simulink model "LinearModelClosedLoopTest_RW_and_Mgt_models"  (R2023a)
settings: Solver=VariableStepAuto  StartTime=0.0  StopTime=500  RelTol=1e-3
values from neighbouring files (symbols this model uses):
  A = [A11 zeros(3) A13 ... (first row only)    [State_Space_SC.m]
  B = (1/438)*(60/(2*pi))*1e-3    (= 2.18020469989e-05)    [State_Space_RW.m]    (also in State_Space_SC.m = [I^-1 I^-1 I^-1)
  I = 1e-7*[336109.715 0 0 ... (first row only)    [State_Space_SC.m]
  J = J_rotor+ J_flywheel    (= 7.1569e-05)    [State_Space_RW.m]
  Ke = (1/1120)*(60/(2*pi))    (= 0.00852615766564)    [State_Space_RW.m]
  Kt = 8.55e-3    (= 0.00855)    [State_Space_RW.m]
  La = 0.222e-3    (= 0.000222)    [State_Space_RW.m]
  Ra = 3.36    [State_Space_RW.m]
  T_ext = 6.850e-7    (= 6.85e-07)    [State_Space_RW.m]
  T_max = 7.7501e-3    (= 0.0077501)    [State_Space_RW.m]
undefined symbols (not defined in the file or in its folder): A_model, B_model, C_model, D_model, n_cal, R_mgt, T_max_mgt
libraries: matrix_library x9, slpidlib x6, simulink_extras x3, vrlib x2, aerolibutil x1
settings Model: Creator=Personal  LastModifiedBy=Personal

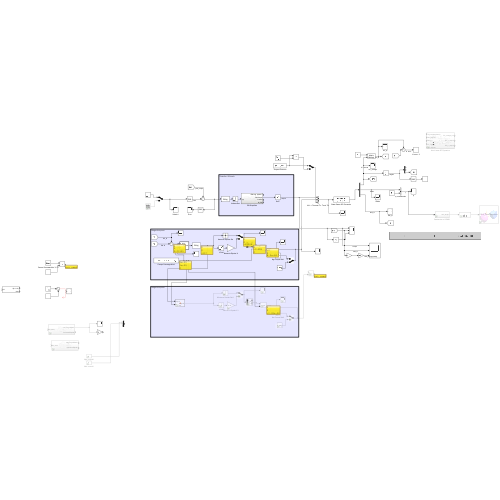
[thumbnail: Simulink's stored preview of the top-level diagram]
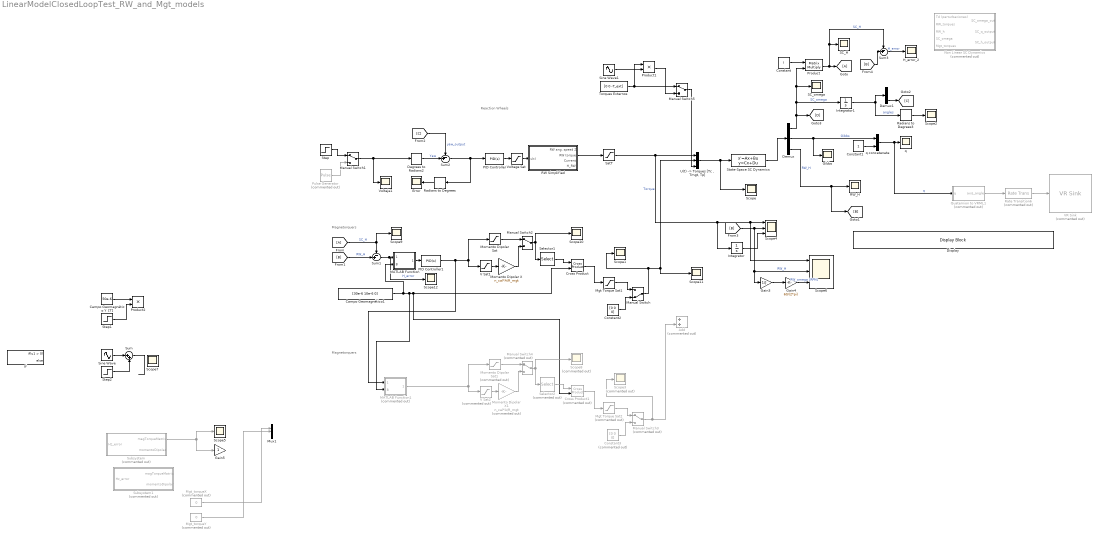
== system LinearModelClosedLoopTest_RW_and_Mgt_models ==
  note: Reaction Wheels
  note: Magnetorquers
  note: Magnetorquers
  Add : Sum  Commented=on
  Campo Geomagnético Y  [T] : Constant  Value=50e-6
  Campo Geomagnético1 : Constant  Value=[30e-6 10e-6 0]
  Constant : Constant  Value=I
  Constant1 : Constant
  Constant2 : Constant  Value=[0 0 0]
  Constant3 : Constant  Commented=on  Value=[0 0 0]
  Cross Product : matrix_library/Cross Product
  Cross Product1 : matrix_library/Cross Product  Commented=on
  Degrees to Radians2 : simulink_extras/Transformations/Degrees to Radians
  Demux : Demux  Outputs=3
  Demux1 : Demux  Outputs=3
  Display : DisplayBlock  LabelPosition=Hide  Transparency=1
  Error : Scope
  From : From
  Gain3 : Gain  Gain=1/J
  Gain4 : Gain  Gain=60/(2*pi)
  Gain5 : Gain
  Gibbs : Scope
  Goto : Goto
  H_error_2 : Scope
  If : If
  Integrator : Integrator
  Integrator1 : Integrator  InitialCondition=[0 0 0]
  MATLAB Function : MATLAB Function  TreatAsAtomicUnit=on
  MATLAB Function1 : MATLAB Function  Commented=on  TreatAsAtomicUnit=on
  Manual Switch : ManualSwitch  CurrentSetting=0
  Manual Switch1 : ManualSwitch
  Manual Switch2 : ManualSwitch
  Manual Switch3 : ManualSwitch  Commented=on
  Manual Switch4 : ManualSwitch  Commented=on
  Manual Switch5 : ManualSwitch
  Mgt Torque Sat1 : Saturate  UpperLimit=T_max_mgt  LowerLimit=-T_max_mgt
  Mgt Torque Sat2 : Saturate  Commented=on  UpperLimit=T_max_mgt  LowerLimit=-T_max_mgt
  Mgt_torqueX : Constant  Commented=on  Value=0
  Mgt_torqueY : Constant  Commented=on  Value=0
  Momento Dipolar Sat : Saturate  UpperLimit=(5/R_mgt)*A*n_cal  LowerLimit=-(5/R_mgt)*A*n_cal
  Momento Dipolar Sat1 : Saturate  Commented=on  UpperLimit=(5/R_mgt)*A*n_cal  LowerLimit=-(5/R_mgt)*A*n_cal
  Momento Dipolar X : Gain  Gain=n_cal*A/R_mgt
  Momento Dipolar X1 : Gain  Commented=on  Gain=n_cal*A/R_mgt
  Mux1 : Mux  Inputs=3
  Non Linear SC Dynamics : Subsystem  Commented=on
  PID Controller : slpidlib/PID Controller  Controller=PID  Form=Parallel  TimeDomain=Continuous-time  UseExternalTs=off  SampleTime=-1  IntegratorMethod=Forward Euler  FilterMethod=Forward Euler  ControllerParametersSource=internal  P=4500  I=800  UseKiTs=off  D=8000  N=100  UseFilter=on  TunerSelectOption=Transfer Function Based (PID Tuner App)  InitialConditionSource=internal  InitialConditionForIntegrator=0  InitialConditionForFilter=0  DifferentiatorICPrevScaledInput=0  ExternalReset=none  TrackingMode=off  Kt=1  LimitOutput=off  SatLimitsSource=internal  UpperSaturationLimit=1  LowerSaturationLimit=-1  LinearizeAsGain=on  AntiWindupMode=none  Kb=1  LimitIntegrator=off  UpperIntegratorSaturationLimit=inf  LowerIntegratorSaturationLimit=-inf  POutMin=[]  POutMax=[]  IOutMin=[]  IOutMax=[]  DOutMin=[]  DOutMax=[]  NOutMin=[]  NOutMax=[]  SumOutMin=[]  SumOutMax=[]  SaturationOutMin=[]  SaturationOutMax=[]  PParamMin=[]  PParamMax=[]  IParamMin=[]  IParamMax=[]  DParamMin=[]  DParamMax=[]  NParamMin=[]  NParamMax=[]  KbParamMin=[]  KbParamMax=[]  KtParamMin=[]  KtParamMax=[]  KbOutMin=[]  KbOutMax=[]  KtOutMin=[]  KtOutMax=[]  IntegratorOutMin=[]  IntegratorOutMax=[]  FilterOutMin=[]  FilterOutMax=[]  SumI1OutMin=[]  SumI1OutMax=[]  SumI2OutMin=[]  SumI2OutMax=[]  SumI3OutMin=[]  SumI3OutMax=[]  SumI4OutMin=[]  SumI4OutMax=[]  SumDOutMin=[]  SumDOutMax=[]  DifferentiatorOutMin=[]  DifferentiatorOutMax=[]  FilterDiffOutCoefMin=[]  FilterDiffOutCoefMax=[]  ReciprocalOutMin=[]  ReciprocalOutMax=[]  SumDenOutMin=[]  SumDenOutMax=[]  SumNumOutMin=[]  SumNumOutMax=[]  DivideOutMin=[]  DivideOutMax=[]  UdiffTsProdOutMin=[]  UdiffTsProdOutMax=[]  NTsProdOutMin=[]  NTsProdOutMax=[]  UintegralTsProdOutMin=[]  UintegralTsProdOutMax=[]  UngainTsProdOutMin=[]  UngainTsProdOutMax=[]  ClampingZeroOutDataTypeStr=Inherit: Inherit via back propagation  ClampingZeroOutMin=[]  ClampingZeroOutMax=[]  FilterDenConstantOutDataTypeStr=Inherit: Inherit via back propagation  FilterDenConstantOutMin=[]  FilterDenConstantOutMax=[]  PCopyOutDataTypeStr=Inherit: Inherit via back propagation  PCopyOutMin=[]  PCopyOutMax=[]  NCopyOutDataTypeStr=Inherit: Inherit via back propagation  NCopyOutMin=[]  NCopyOutMax=[]  IntegratorContinuousStateAttributes=''  IntegratorStateMustResolveToSignalObject=off  IntegratorRTWStateStorageClass=Auto  FilterContinuousStateAttributes=''  FilterStateMustResolveToSignalObject=off  FilterRTWStateStorageClass=Auto  ParallelPVariant=InternalParameters  IdealPVariant=Disabled  IVariant=InternalParameters  DVariant=InternalParameters  IntegratorVariant=Continuous  SatVariant=Disabled  AWVariant=Passthrough  PCopyVariant=Disabled  TRVariant=Disabled  FdbkBlocksVariant=Forward  IdealPFdbkVariant=Disabled  SatFdbkVariant=Disabled  DerivativeFilterVariant=ContFilter  NVariant=InternalParameters  NCopyVariant=Disabled  FilterICVariant=InternalICsFilter  IntegratorICVariant=InternalICs  ExternalResetVariant=Disabled  TRSumVariant=Passthrough  SumFdbkVariant=Disabled  SumVariant=Sum_PID  TsampFilterVariant=InternalTs  TsampNgainVariant=Passthrough  TsampIntegralVariant=Disabled_SignalSpec  ExternalSaturationOutDataTypeStr=Inherit: Same as second input
  PID Controller1 : slpidlib/PID Controller  Controller=PID  Form=Parallel  TimeDomain=Continuous-time  UseExternalTs=off  SampleTime=-1  IntegratorMethod=Forward Euler  FilterMethod=Forward Euler  ControllerParametersSource=internal  P=4500  I=800  UseKiTs=off  D=8000  N=100  UseFilter=on  TunerSelectOption=Transfer Function Based (PID Tuner App)  InitialConditionSource=internal  InitialConditionForIntegrator=0  InitialConditionForFilter=0  DifferentiatorICPrevScaledInput=0  ExternalReset=none  TrackingMode=off  Kt=1  LimitOutput=off  SatLimitsSource=internal  UpperSaturationLimit=1  LowerSaturationLimit=-1  LinearizeAsGain=on  AntiWindupMode=none  Kb=1  LimitIntegrator=off  UpperIntegratorSaturationLimit=inf  LowerIntegratorSaturationLimit=-inf  POutMin=[]  POutMax=[]  IOutMin=[]  IOutMax=[]  DOutMin=[]  DOutMax=[]  NOutMin=[]  NOutMax=[]  SumOutMin=[]  SumOutMax=[]  SaturationOutMin=[]  SaturationOutMax=[]  PParamMin=[]  PParamMax=[]  IParamMin=[]  IParamMax=[]  DParamMin=[]  DParamMax=[]  NParamMin=[]  NParamMax=[]  KbParamMin=[]  KbParamMax=[]  KtParamMin=[]  KtParamMax=[]  KbOutMin=[]  KbOutMax=[]  KtOutMin=[]  KtOutMax=[]  IntegratorOutMin=[]  IntegratorOutMax=[]  FilterOutMin=[]  FilterOutMax=[]  SumI1OutMin=[]  SumI1OutMax=[]  SumI2OutMin=[]  SumI2OutMax=[]  SumI3OutMin=[]  SumI3OutMax=[]  SumI4OutMin=[]  SumI4OutMax=[]  SumDOutMin=[]  SumDOutMax=[]  DifferentiatorOutMin=[]  DifferentiatorOutMax=[]  FilterDiffOutCoefMin=[]  FilterDiffOutCoefMax=[]  ReciprocalOutMin=[]  ReciprocalOutMax=[]  SumDenOutMin=[]  SumDenOutMax=[]  SumNumOutMin=[]  SumNumOutMax=[]  DivideOutMin=[]  DivideOutMax=[]  UdiffTsProdOutMin=[]  UdiffTsProdOutMax=[]  NTsProdOutMin=[]  NTsProdOutMax=[]  UintegralTsProdOutMin=[]  UintegralTsProdOutMax=[]  UngainTsProdOutMin=[]  UngainTsProdOutMax=[]  ClampingZeroOutDataTypeStr=Inherit: Inherit via back propagation  ClampingZeroOutMin=[]  ClampingZeroOutMax=[]  FilterDenConstantOutDataTypeStr=Inherit: Inherit via back propagation  FilterDenConstantOutMin=[]  FilterDenConstantOutMax=[]  PCopyOutDataTypeStr=Inherit: Inherit via back propagation  PCopyOutMin=[]  PCopyOutMax=[]  NCopyOutDataTypeStr=Inherit: Inherit via back propagation  NCopyOutMin=[]  NCopyOutMax=[]  IntegratorContinuousStateAttributes=''  IntegratorStateMustResolveToSignalObject=off  IntegratorRTWStateStorageClass=Auto  FilterContinuousStateAttributes=''  FilterStateMustResolveToSignalObject=off  FilterRTWStateStorageClass=Auto  ParallelPVariant=InternalParameters  IdealPVariant=Disabled  IVariant=InternalParameters  DVariant=InternalParameters  IntegratorVariant=Continuous  SatVariant=Disabled  AWVariant=Passthrough  PCopyVariant=Disabled  TRVariant=Disabled  FdbkBlocksVariant=Forward  IdealPFdbkVariant=Disabled  SatFdbkVariant=Disabled  DerivativeFilterVariant=ContFilter  NVariant=InternalParameters  NCopyVariant=Disabled  FilterICVariant=InternalICsFilter  IntegratorICVariant=InternalICs  ExternalResetVariant=Disabled  TRSumVariant=Passthrough  SumFdbkVariant=Disabled  SumVariant=Sum_PID  TsampFilterVariant=InternalTs  TsampNgainVariant=Passthrough  TsampIntegralVariant=Disabled_SignalSpec  ExternalSaturationOutDataTypeStr=Inherit: Same as second input
  Product : Product  Multiplication=Matrix(*)
  Product1 : Product
  Product2 : Product
  Pulse Generator : DiscretePulseGenerator  Commented=on  PulseType=Time based  Amplitude=45  Period=50  PulseWidth=50
  Quaternion to VRML1 : Subsystem  Commented=on
  RW Simplified : Subsystem
  RW_H : Scope
  Radians to Degrees : simulink_extras/Transformations/Radians to Degrees
  Radians to Degrees3 : simulink_extras/Transformations/Radians to Degrees
  Rate Transition6 : RateTransition  Commented=on
  SC_H : Scope
  SC_omega : Scope
  SatT : Saturate  UpperLimit=T_max  LowerLimit=-T_max
  Scope{,1..2,5,7,9..12} (9 alike) : Scope
  Scope3 : Scope  Commented=on
  Scope4 : Scope  NumInputPorts=3
  Scope6 : Scope  NumInputPorts=3
  Scope8 : Scope  Commented=on
  Selector1 : Selector  InputPortWidth=3  IndexOptions=Index vector (dialog)  Indices=[1 3 2]  OutputSizes=1
  Selector2 : Selector  Commented=on  InputPortWidth=3  IndexOptions=Index vector (dialog)  Indices=[3 1 2]  OutputSizes=1
  Sine Wave : Sin  Amplitude=3e-6  Frequency=0.1  SampleTime=0
  Sine Wave1 : Sin  Frequency=0.05  SampleTime=0
  "State-Space SC Dynamics " : StateSpace  A=A_model  B=B_model  C=C_model  D=D_model  InitialCondition=0
  Step : Step  Time=5  After=90  SampleTime=0
  Step1 : Step  Time=0  SampleTime=0
  Step2 : Step  Time=0  After=40e-6  SampleTime=0
  Subsystem : Subsystem  Commented=on
  Subsystem1 : Subsystem  Commented=on
  Sum : Sum  Inputs=|++
  Sum1 : Sum  Inputs=-+|
  Sum2 : Sum  Inputs=-+|
  Sum3 : Sum  Inputs=-+|
  Torques Externos : Constant  Value=[0 0 -T_ext]
  "U(t) -> Torques [Tc , Tmgt, Tp]" : Concatenate  NumInputs=3
  V Sat1 : Saturate  UpperLimit=5  LowerLimit=-5
  V Sat2 : Saturate  Commented=on  UpperLimit=5  LowerLimit=-5
  VR Sink : vrlib/VR Sink  Commented=on  InstantiateOnLoad=on  SampleTime=0.1  ViewEnable=on  RemoteChange=off  RemoteView=off  FieldsWritten=STLB_Transform.rotation.4.1.1.double  WorldFileName=EscenarioCubeSat.x3d  AutoView=off  VideoDimensions=[]  AllowVariableSize=off
  Voltage Sat : Saturate  UpperLimit=6  LowerLimit=-6
  Voltaje1 : Scope
  q : Scope
  q concatenate : Concatenate
  wires:
  Pulse Generator/1 -> Manual Switch1/2
  Degrees to Radians2/1 -> Sum2/2  "Yaw"
  Manual Switch1/1 -> Voltaje1/1, Degrees to Radians2/1
  Step/1 -> Manual Switch1/1
  "State-Space SC Dynamics "/1 -> Demux/1
  "U(t) -> Torques [Tc , Tmgt, Tp]"/1 -> Scope/1, "State-Space SC Dynamics "/1
  Demux/1 -> [D], Integrator1/1, Product/2, SC_omega/1  "SC_omega"
  Demux/2 -> q concatenate/1, Gibbs/1  "Gibbs"
  Demux/3 -> [B], RW_H/1  "RW_H"
  Sum2/1 -> Radians to Degrees/1, PID Controller/1
  SatT/1 -> Integrator/1, Scope6/1, Scope4/1, "U(t) -> Torques [Tc , Tmgt, Tp]"/1  "Torque"
  Torques Externos/1 -> Product1/1, Manual Switch5/1
  Subsystem/1(magTorqueMatrix) -> Scope5/1, Gain5/1
  Constant/1 -> Product/1
  Product/1 -> Sum3/1, SC_H/1, Goto/1  "SC_H"
  From/1 -> Sum1/1, Scope9/1  "SC_H"
  [B] -> Sum1/2  "RW_H"
  Sum1/1 -> Scope12/1, MATLAB Function/1("H_error ")  "H_error"
  Integrator1/1 -> Demux1/1, Radians to Degrees3/1  "angles"
  Demux1/3 -> [C]
  Radians to Degrees3/1 -> Scope2/1
  [C] -> Sum2/1  "yaw_output"
  Radians to Degrees/1 -> Error/1
  [B] -> Gain3/1, Scope6/2, Scope4/2  "RW_H"
  Integrator/1 -> Scope4/3
  Constant1/1 -> q concatenate/2
  q concatenate/1 -> Quaternion to VRML1/1(q), q/1  "q"
  Rate Transition6/1 -> VR Sink/1
  Quaternion to VRML1/1(axis_angle) -> Rate Transition6/1
  Gain3/1 -> Gain4/1
  Gain4/1 -> Scope6/3  "RW_omega [RPM]"
  RW Simplified/2(RW torque) -> SatT/1
  PID Controller/1 -> Voltage Sat/1
  Voltage Sat/1 -> RW Simplified/1(v(t))
  Mgt_torqueY/1 -> Mux1/2
  Mgt_torqueX/1 -> Mux1/1
  Mgt Torque Sat1/1 -> Manual Switch/1
  [B] -> Sum3/2
  Sum3/1 -> H_error_2/1  "H_error"
  V Sat1/1 -> Momento Dipolar X/1
  Momento Dipolar X/1 -> Manual Switch2/2
  Campo Geomagnético Y  [T]/1 -> Product2/1
  Step1/1 -> Product2/2
  Sine Wave/1 -> Sum/1
  Step2/1 -> Sum/2
  Sum/1 -> ?
  Momento Dipolar Sat/1 -> Manual Switch2/1
  MATLAB Function/1(H_error) -> PID Controller1/1
  Manual Switch2/1 -> Selector1/1, Scope10/1
  Campo Geomagnético1/1 -> MATLAB Function1/2(B), Cross Product1/2, Cross Product/2, MATLAB Function/2(B)
  Manual Switch/1 -> "U(t) -> Torques [Tc , Tmgt, Tp]"/2, Scope11/1, Scope1/1
  Selector1/1 -> Cross Product/1
  Cross Product/1 -> Mgt Torque Sat1/1
  PID Controller1/1 -> MATLAB Function1/1("signal "), Momento Dipolar Sat/1, V Sat1/1
  Constant2/1 -> Manual Switch/2
  Constant3/1 -> Manual Switch3/2
  MATLAB Function1/1(signal) -> V Sat2/1, Momento Dipolar Sat1/1
  Cross Product1/1 -> Mgt Torque Sat2/1
  Selector2/1 -> Cross Product1/1
  Manual Switch3/1 -> Scope3/1, Add/2
  Manual Switch4/1 -> Scope8/1, Selector2/1
  Momento Dipolar Sat1/1 -> Manual Switch4/1
  Momento Dipolar X1/1 -> Manual Switch4/2
  V Sat2/1 -> Momento Dipolar X1/1
  Mgt Torque Sat2/1 -> Manual Switch3/1
  Sine Wave1/1 -> Product1/2
  Manual Switch5/1 -> "U(t) -> Torques [Tc , Tmgt, Tp]"/3
  Product1/1 -> Manual Switch5/2

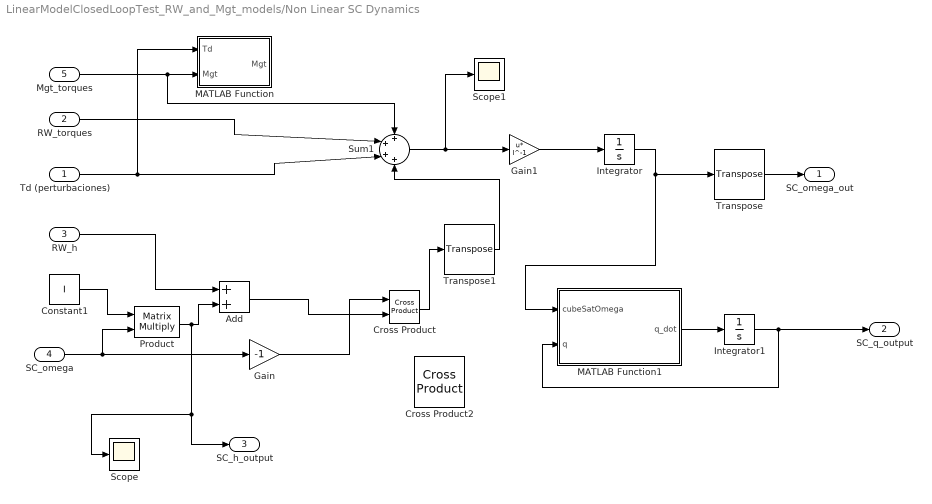
== system LinearModelClosedLoopTest_RW_and_Mgt_models/Non Linear SC Dynamics ==
  Td (perturbaciones) : Inport
  RW_torques : Inport  Port=2
  RW_h : Inport  Port=3
  SC_omega : Inport  Port=4
  Mgt_torques : Inport  Port=5
  Add : Sum
  Constant1 : Constant  Value=I
  Cross Product : vrlib/Utilities/Cross Product
  Cross Product2 : matrix_library/Cross Product
  Gain : Gain  Gain=-1
  Gain1 : Gain  Gain=I^-1  Multiplication=Matrix(u*K)
  Integrator : Integrator  InitialCondition=[0 0 0]
  Integrator1 : Integrator  InitialCondition=[0 0 0 1]
  MATLAB Function : MATLAB Function  TreatAsAtomicUnit=on
  MATLAB Function1 : MATLAB Function  TreatAsAtomicUnit=on
  Product : Product  Multiplication=Matrix(*)
  Scope : Scope
  Scope1 : Scope
  Sum1 : Sum  Inputs=++++
  Transpose : matrix_library/Transpose
  Transpose1 : matrix_library/Transpose
  SC_omega_out : Outport
  SC_q_output : Outport  Port=2
  SC_h_output : Outport  Port=3
  wires:
  RW_torques/1 -> Sum1/2
  Td (perturbaciones)/1 -> MATLAB Function/1(Td), Sum1/3
  Integrator1/1 -> MATLAB Function1/2(q), SC_q_output/1
  Constant1/1 -> Product/1
  Product/1 -> Scope/1, SC_h_output/1, Add/2
  RW_h/1 -> Add/1
  Gain/1 -> Cross Product/1
  Add/1 -> Cross Product/2
  Cross Product/1 -> Transpose1/1
  Sum1/1 -> Scope1/1, Gain1/1
  Gain1/1 -> Integrator/1
  Integrator/1 -> MATLAB Function1/1(cubeSatOmega), Transpose/1
  MATLAB Function1/1(q_dot) -> Integrator1/1
  SC_omega/1 -> Product/2, Gain/1
  Transpose/1 -> SC_omega_out/1
  Transpose1/1 -> Sum1/4
  Mgt_torques/1 -> Sum1/1, MATLAB Function/2("Mgt ")

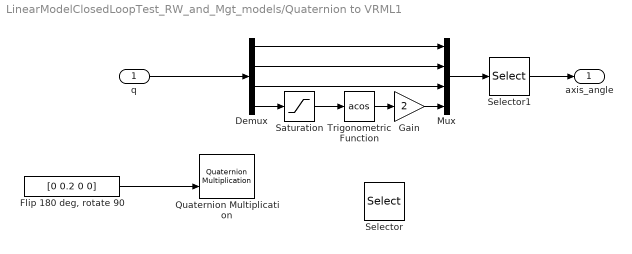
== system LinearModelClosedLoopTest_RW_and_Mgt_models/Quaternion to VRML1 ==
  q : Inport
  Demux : Demux
  "Flip 180 deg, rotate 90" : Constant  Value=[0 0.2 0 0]
  Gain : Gain  Gain=2
  Mux : Mux
  Quaternion Multiplication : aerolibutil/Quaternion Multiplication
  Saturation : Saturate  UpperLimit=1  LowerLimit=-1  ZeroCross=off
  Selector : Selector  InputPortWidth=3  IndexOptions=Index vector (dialog)  Indices=[1 3]  OutputSizes=1
  Selector1 : Selector  InputPortWidth=4  IndexOptions=Index vector (dialog)  Indices=[2 3 1 4]  OutputSizes=1
  Trigonometric Function : Trigonometry  Operator=acos
  axis_angle : Outport  VectorParamsAs1DForOutWhenUnconnected=off
  wires:
  Demux/2 -> Mux/2
  "Flip 180 deg, rotate 90"/1 -> Quaternion Multiplication/2
  q/1 -> Demux/1
  Demux/1 -> Mux/1
  Mux/1 -> Selector1/1
  Selector1/1 -> axis_angle/1
  Trigonometric Function/1 -> Gain/1
  Gain/1 -> Mux/4
  Demux/3 -> Mux/3
  Saturation/1 -> Trigonometric Function/1
  Demux/4 -> Saturation/1

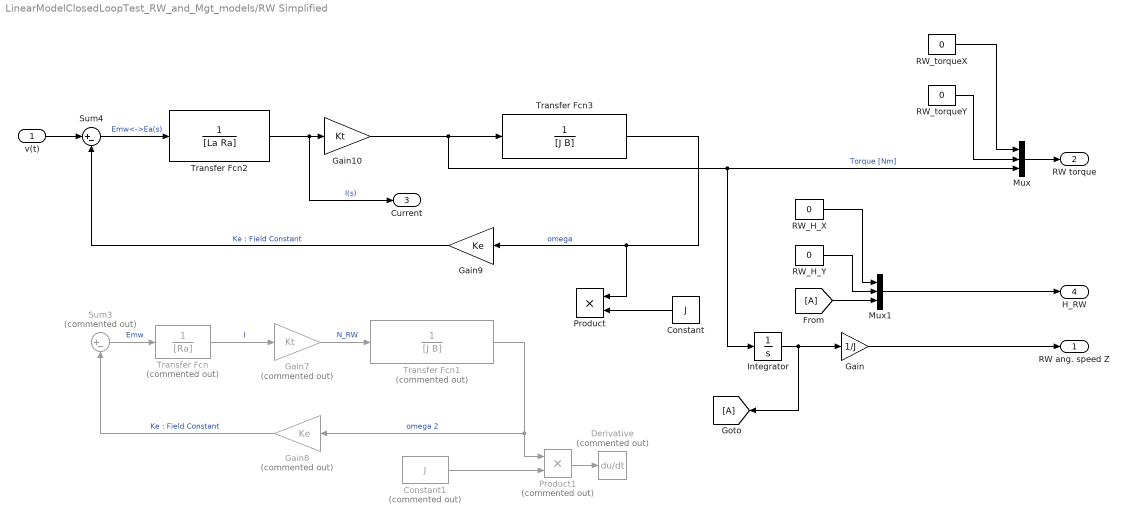
== system LinearModelClosedLoopTest_RW_and_Mgt_models/RW Simplified ==
  v(t) : Inport
  Constant : Constant  Value=J
  Constant1 : Constant  Commented=on  Value=J
  Derivative : Derivative  Commented=on
  From : From
  Gain : Gain  Gain=1/J
  Gain10 : Gain  Gain=Kt
  Gain7 : Gain  Commented=on  Gain=Kt
  Gain8 : Gain  Commented=on  Gain=Ke
  Gain9 : Gain  Gain=Ke
  Goto : Goto
  Integrator : Integrator
  Mux : Mux  Inputs=3
  Mux1 : Mux  Inputs=3
  Product : Product
  Product1 : Product  Commented=on
  RW_H_X : Constant  Value=0
  RW_H_Y : Constant  Value=0
  RW_torqueX : Constant  Value=0
  RW_torqueY : Constant  Value=0
  Sum3 : Sum  Commented=on  Inputs=|+-
  Sum4 : Sum  Inputs=|+-
  Transfer Fcn : TransferFcn  Commented=on  Denominator=[Ra]
  Transfer Fcn1 : TransferFcn  Commented=on  Denominator=[J B]
  Transfer Fcn2 : TransferFcn  Denominator=[La Ra]
  Transfer Fcn3 : TransferFcn  Denominator=[J B]
  RW ang. speed Z : Outport  VectorParamsAs1DForOutWhenUnconnected=off
  RW torque : Outport  Port=2  VectorParamsAs1DForOutWhenUnconnected=off
  Current : Outport  Port=3  VectorParamsAs1DForOutWhenUnconnected=off
  H_RW : Outport  Port=4  VectorParamsAs1DForOutWhenUnconnected=off
  wires:
  Transfer Fcn2/1 -> Current/1, Gain10/1  "I(s)"
  Sum4/1 -> Transfer Fcn2/1  "Emw<->Ea(s)"
  Gain9/1 -> Sum4/2  "Ke : Field Constant"
  Transfer Fcn3/1 -> Gain9/1, Product/1  "omega"
  Constant/1 -> Product/2
  Integrator/1 -> Goto/1, Gain/1
  v(t)/1 -> Sum4/1
  Product1/1 -> Derivative/1
  Constant1/1 -> Product1/2
  Transfer Fcn1/1 -> Product1/1, Gain8/1  "omega 2"
  Gain7/1 -> Transfer Fcn1/1  "N_RW"
  Sum3/1 -> Transfer Fcn/1  "Emw"
  Transfer Fcn/1 -> Gain7/1  "I"
  Gain8/1 -> Sum3/2  "Ke : Field Constant"
  RW_H_X/1 -> Mux1/1
  RW_H_Y/1 -> Mux1/2
  Mux1/1 -> H_RW/1
  RW_torqueX/1 -> Mux/1
  RW_torqueY/1 -> Mux/2
  Mux/1 -> RW torque/1
  Gain10/1 -> Integrator/1, Mux/3, Transfer Fcn3/1  "Torque [Nm]"
  Gain/1 -> RW ang. speed Z/1
  From/1 -> Mux1/3

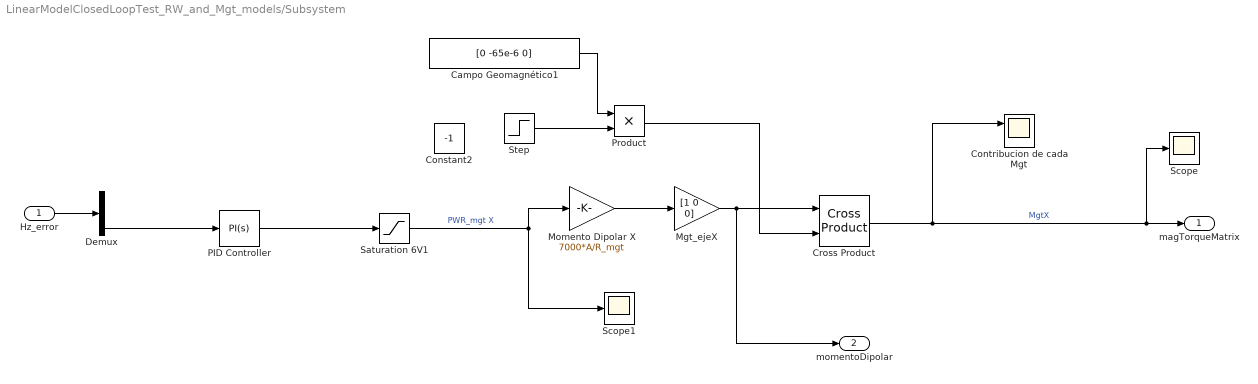
== system LinearModelClosedLoopTest_RW_and_Mgt_models/Subsystem ==
  Hz_error : Inport
  Campo Geomagnético1 : Constant  Value=[0 -65e-6 0]
  Constant2 : Constant  Value=-1
  Contribucion de cada Mgt : Scope  NumInputPorts=2
  Cross Product : matrix_library/Cross Product
  Demux : Demux  Outputs=3
  Mgt_ejeX : Gain  Gain=[1 0 0]
  Momento Dipolar X : Gain  Gain=7000*A/R_mgt
  PID Controller : slpidlib/PID Controller  Controller=PI  Form=Parallel  TimeDomain=Continuous-time  UseExternalTs=off  SampleTime=-1  IntegratorMethod=Forward Euler  FilterMethod=Forward Euler  ControllerParametersSource=internal  P=1  I=1  UseKiTs=off  D=0  N=100  UseFilter=on  TunerSelectOption=Transfer Function Based (PID Tuner App)  InitialConditionSource=internal  InitialConditionForIntegrator=0  InitialConditionForFilter=0  DifferentiatorICPrevScaledInput=0  ExternalReset=none  TrackingMode=off  Kt=1  LimitOutput=off  SatLimitsSource=internal  UpperSaturationLimit=inf  LowerSaturationLimit=-inf  LinearizeAsGain=on  AntiWindupMode=none  Kb=1  LimitIntegrator=off  UpperIntegratorSaturationLimit=inf  LowerIntegratorSaturationLimit=-inf  POutMin=[]  POutMax=[]  IOutMin=[]  IOutMax=[]  DOutMin=[]  DOutMax=[]  NOutMin=[]  NOutMax=[]  SumOutMin=[]  SumOutMax=[]  SaturationOutMin=[]  SaturationOutMax=[]  PParamMin=[]  PParamMax=[]  IParamMin=[]  IParamMax=[]  DParamMin=[]  DParamMax=[]  NParamMin=[]  NParamMax=[]  KbParamMin=[]  KbParamMax=[]  KtParamMin=[]  KtParamMax=[]  KbOutMin=[]  KbOutMax=[]  KtOutMin=[]  KtOutMax=[]  IntegratorOutMin=[]  IntegratorOutMax=[]  FilterOutMin=[]  FilterOutMax=[]  SumI1OutMin=[]  SumI1OutMax=[]  SumI2OutMin=[]  SumI2OutMax=[]  SumI3OutMin=[]  SumI3OutMax=[]  SumI4OutMin=[]  SumI4OutMax=[]  SumDOutMin=[]  SumDOutMax=[]  DifferentiatorOutMin=[]  DifferentiatorOutMax=[]  FilterDiffOutCoefMin=[]  FilterDiffOutCoefMax=[]  ReciprocalOutMin=[]  ReciprocalOutMax=[]  SumDenOutMin=[]  SumDenOutMax=[]  SumNumOutMin=[]  SumNumOutMax=[]  DivideOutMin=[]  DivideOutMax=[]  UdiffTsProdOutMin=[]  UdiffTsProdOutMax=[]  NTsProdOutMin=[]  NTsProdOutMax=[]  UintegralTsProdOutMin=[]  UintegralTsProdOutMax=[]  UngainTsProdOutMin=[]  UngainTsProdOutMax=[]  ClampingZeroOutDataTypeStr=Inherit: Inherit via back propagation  ClampingZeroOutMin=[]  ClampingZeroOutMax=[]  FilterDenConstantOutDataTypeStr=Inherit: Inherit via back propagation  FilterDenConstantOutMin=[]  FilterDenConstantOutMax=[]  PCopyOutDataTypeStr=Inherit: Inherit via back propagation  PCopyOutMin=[]  PCopyOutMax=[]  NCopyOutDataTypeStr=Inherit: Inherit via back propagation  NCopyOutMin=[]  NCopyOutMax=[]  IntegratorContinuousStateAttributes=''  IntegratorStateMustResolveToSignalObject=off  IntegratorRTWStateStorageClass=Auto  FilterContinuousStateAttributes=''  FilterStateMustResolveToSignalObject=off  FilterRTWStateStorageClass=Auto  ParallelPVariant=InternalParameters  IdealPVariant=Disabled  IVariant=InternalParameters  DVariant=Disabled  IntegratorVariant=Continuous  SatVariant=Disabled  AWVariant=Passthrough  PCopyVariant=Disabled  TRVariant=Disabled  FdbkBlocksVariant=Forward  IdealPFdbkVariant=Disabled  SatFdbkVariant=Disabled  DerivativeFilterVariant=Disabled  NVariant=Disabled  NCopyVariant=Disabled_SignalSpec  FilterICVariant=Disabled  IntegratorICVariant=InternalICs  ExternalResetVariant=Disabled  TRSumVariant=Passthrough  SumFdbkVariant=Disabled  SumVariant=Sum_PI  TsampFilterVariant=InternalTs  TsampNgainVariant=Passthrough  TsampIntegralVariant=Disabled_SignalSpec  ExternalSaturationOutDataTypeStr=Inherit: Same as second input
  Product : Product
  Saturation 6V1 : Saturate  UpperLimit=10  LowerLimit=-10
  Scope : Scope
  Scope1 : Scope
  Step : Step  Time=0  After=-1  SampleTime=0
  magTorqueMatrix : Outport
  momentoDipolar : Outport  Port=2
  wires:
  Saturation 6V1/1 -> Momento Dipolar X/1, Scope1/1  "PWR_mgt X"
  Hz_error/1 -> Demux/1
  Product/1 -> Cross Product/2
  PID Controller/1 -> Saturation 6V1/1
  Momento Dipolar X/1 -> Mgt_ejeX/1
  Cross Product/1 -> Contribucion de cada Mgt/1, Scope/1, magTorqueMatrix/1  "MgtX"
  Mgt_ejeX/1 -> momentoDipolar/1, Cross Product/1
  Campo Geomagnético1/1 -> Product/1
  Step/1 -> Product/2
  Demux/3 -> PID Controller/1

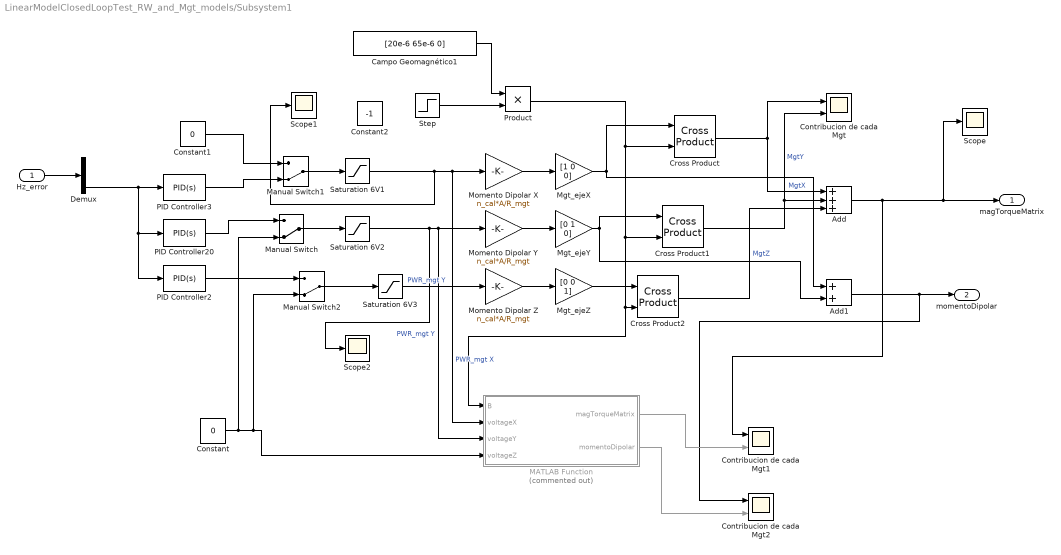
== system LinearModelClosedLoopTest_RW_and_Mgt_models/Subsystem1 ==
  Hz_error : Inport
  Add : Sum  Inputs=+++
  Add1 : Sum
  Campo Geomagnético1 : Constant  Value=[20e-6 65e-6 0]
  Constant : Constant  Value=0
  Constant1 : Constant  Value=0
  Constant2 : Constant  Value=-1
  Contribucion de cada Mgt : Scope  NumInputPorts=2
  Contribucion de cada Mgt1 : Scope  NumInputPorts=2
  Contribucion de cada Mgt2 : Scope  NumInputPorts=2
  Cross Product : matrix_library/Cross Product
  Cross Product1 : matrix_library/Cross Product
  Cross Product2 : matrix_library/Cross Product
  Demux : Demux  Outputs=3
  MATLAB Function : MATLAB Function  Commented=on  TreatAsAtomicUnit=on
  Manual Switch : ManualSwitch  CurrentSetting=0
  Manual Switch1 : ManualSwitch  CurrentSetting=0
  Manual Switch2 : ManualSwitch  CurrentSetting=0
  Mgt_ejeX : Gain  Gain=[1 0 0]
  Mgt_ejeY : Gain  Gain=[0 1 0]
  Mgt_ejeZ : Gain  Gain=[0 0 1]
  Momento Dipolar X : Gain  Gain=n_cal*A/R_mgt
  Momento Dipolar Y : Gain  Gain=n_cal*A/R_mgt
  Momento Dipolar Z : Gain  Gain=n_cal*A/R_mgt
  PID Controller2 : slpidlib/PID Controller  Controller=PID  Form=Parallel  TimeDomain=Continuous-time  UseExternalTs=off  SampleTime=-1  IntegratorMethod=Forward Euler  FilterMethod=Forward Euler  ControllerParametersSource=internal  P=4500  I=800  UseKiTs=off  D=8000  N=100  UseFilter=on  TunerSelectOption=Transfer Function Based (PID Tuner App)  InitialConditionSource=internal  InitialConditionForIntegrator=0  InitialConditionForFilter=0  DifferentiatorICPrevScaledInput=0  ExternalReset=none  TrackingMode=off  Kt=1  LimitOutput=off  SatLimitsSource=internal  UpperSaturationLimit=1  LowerSaturationLimit=-1  LinearizeAsGain=on  AntiWindupMode=none  Kb=1  LimitIntegrator=off  UpperIntegratorSaturationLimit=inf  LowerIntegratorSaturationLimit=-inf  POutMin=[]  POutMax=[]  IOutMin=[]  IOutMax=[]  DOutMin=[]  DOutMax=[]  NOutMin=[]  NOutMax=[]  SumOutMin=[]  SumOutMax=[]  SaturationOutMin=[]  SaturationOutMax=[]  PParamMin=[]  PParamMax=[]  IParamMin=[]  IParamMax=[]  DParamMin=[]  DParamMax=[]  NParamMin=[]  NParamMax=[]  KbParamMin=[]  KbParamMax=[]  KtParamMin=[]  KtParamMax=[]  KbOutMin=[]  KbOutMax=[]  KtOutMin=[]  KtOutMax=[]  IntegratorOutMin=[]  IntegratorOutMax=[]  FilterOutMin=[]  FilterOutMax=[]  SumI1OutMin=[]  SumI1OutMax=[]  SumI2OutMin=[]  SumI2OutMax=[]  SumI3OutMin=[]  SumI3OutMax=[]  SumI4OutMin=[]  SumI4OutMax=[]  SumDOutMin=[]  SumDOutMax=[]  DifferentiatorOutMin=[]  DifferentiatorOutMax=[]  FilterDiffOutCoefMin=[]  FilterDiffOutCoefMax=[]  ReciprocalOutMin=[]  ReciprocalOutMax=[]  SumDenOutMin=[]  SumDenOutMax=[]  SumNumOutMin=[]  SumNumOutMax=[]  DivideOutMin=[]  DivideOutMax=[]  UdiffTsProdOutMin=[]  UdiffTsProdOutMax=[]  NTsProdOutMin=[]  NTsProdOutMax=[]  UintegralTsProdOutMin=[]  UintegralTsProdOutMax=[]  UngainTsProdOutMin=[]  UngainTsProdOutMax=[]  ClampingZeroOutDataTypeStr=Inherit: Inherit via back propagation  ClampingZeroOutMin=[]  ClampingZeroOutMax=[]  FilterDenConstantOutDataTypeStr=Inherit: Inherit via back propagation  FilterDenConstantOutMin=[]  FilterDenConstantOutMax=[]  PCopyOutDataTypeStr=Inherit: Inherit via back propagation  PCopyOutMin=[]  PCopyOutMax=[]  NCopyOutDataTypeStr=Inherit: Inherit via back propagation  NCopyOutMin=[]  NCopyOutMax=[]  IntegratorContinuousStateAttributes=''  IntegratorStateMustResolveToSignalObject=off  IntegratorRTWStateStorageClass=Auto  FilterContinuousStateAttributes=''  FilterStateMustResolveToSignalObject=off  FilterRTWStateStorageClass=Auto  ParallelPVariant=InternalParameters  IdealPVariant=Disabled  IVariant=InternalParameters  DVariant=InternalParameters  IntegratorVariant=Continuous  SatVariant=Disabled  AWVariant=Passthrough  PCopyVariant=Disabled  TRVariant=Disabled  FdbkBlocksVariant=Forward  IdealPFdbkVariant=Disabled  SatFdbkVariant=Disabled  DerivativeFilterVariant=ContFilter  NVariant=InternalParameters  NCopyVariant=Disabled  FilterICVariant=InternalICsFilter  IntegratorICVariant=InternalICs  ExternalResetVariant=Disabled  TRSumVariant=Passthrough  SumFdbkVariant=Disabled  SumVariant=Sum_PID  TsampFilterVariant=InternalTs  TsampNgainVariant=Passthrough  TsampIntegralVariant=Disabled_SignalSpec  ExternalSaturationOutDataTypeStr=Inherit: Same as second input
  PID Controller20 : slpidlib/PID Controller  Controller=PID  Form=Parallel  TimeDomain=Continuous-time  UseExternalTs=off  SampleTime=-1  IntegratorMethod=Forward Euler  FilterMethod=Forward Euler  ControllerParametersSource=internal  P=4500  I=800  UseKiTs=off  D=8000  N=100  UseFilter=on  TunerSelectOption=Transfer Function Based (PID Tuner App)  InitialConditionSource=internal  InitialConditionForIntegrator=0  InitialConditionForFilter=0  DifferentiatorICPrevScaledInput=0  ExternalReset=none  TrackingMode=off  Kt=1  LimitOutput=off  SatLimitsSource=internal  UpperSaturationLimit=1  LowerSaturationLimit=-1  LinearizeAsGain=on  AntiWindupMode=none  Kb=1  LimitIntegrator=off  UpperIntegratorSaturationLimit=inf  LowerIntegratorSaturationLimit=-inf  POutMin=[]  POutMax=[]  IOutMin=[]  IOutMax=[]  DOutMin=[]  DOutMax=[]  NOutMin=[]  NOutMax=[]  SumOutMin=[]  SumOutMax=[]  SaturationOutMin=[]  SaturationOutMax=[]  PParamMin=[]  PParamMax=[]  IParamMin=[]  IParamMax=[]  DParamMin=[]  DParamMax=[]  NParamMin=[]  NParamMax=[]  KbParamMin=[]  KbParamMax=[]  KtParamMin=[]  KtParamMax=[]  KbOutMin=[]  KbOutMax=[]  KtOutMin=[]  KtOutMax=[]  IntegratorOutMin=[]  IntegratorOutMax=[]  FilterOutMin=[]  FilterOutMax=[]  SumI1OutMin=[]  SumI1OutMax=[]  SumI2OutMin=[]  SumI2OutMax=[]  SumI3OutMin=[]  SumI3OutMax=[]  SumI4OutMin=[]  SumI4OutMax=[]  SumDOutMin=[]  SumDOutMax=[]  DifferentiatorOutMin=[]  DifferentiatorOutMax=[]  FilterDiffOutCoefMin=[]  FilterDiffOutCoefMax=[]  ReciprocalOutMin=[]  ReciprocalOutMax=[]  SumDenOutMin=[]  SumDenOutMax=[]  SumNumOutMin=[]  SumNumOutMax=[]  DivideOutMin=[]  DivideOutMax=[]  UdiffTsProdOutMin=[]  UdiffTsProdOutMax=[]  NTsProdOutMin=[]  NTsProdOutMax=[]  UintegralTsProdOutMin=[]  UintegralTsProdOutMax=[]  UngainTsProdOutMin=[]  UngainTsProdOutMax=[]  ClampingZeroOutDataTypeStr=Inherit: Inherit via back propagation  ClampingZeroOutMin=[]  ClampingZeroOutMax=[]  FilterDenConstantOutDataTypeStr=Inherit: Inherit via back propagation  FilterDenConstantOutMin=[]  FilterDenConstantOutMax=[]  PCopyOutDataTypeStr=Inherit: Inherit via back propagation  PCopyOutMin=[]  PCopyOutMax=[]  NCopyOutDataTypeStr=Inherit: Inherit via back propagation  NCopyOutMin=[]  NCopyOutMax=[]  IntegratorContinuousStateAttributes=''  IntegratorStateMustResolveToSignalObject=off  IntegratorRTWStateStorageClass=Auto  FilterContinuousStateAttributes=''  FilterStateMustResolveToSignalObject=off  FilterRTWStateStorageClass=Auto  ParallelPVariant=InternalParameters  IdealPVariant=Disabled  IVariant=InternalParameters  DVariant=InternalParameters  IntegratorVariant=Continuous  SatVariant=Disabled  AWVariant=Passthrough  PCopyVariant=Disabled  TRVariant=Disabled  FdbkBlocksVariant=Forward  IdealPFdbkVariant=Disabled  SatFdbkVariant=Disabled  DerivativeFilterVariant=ContFilter  NVariant=InternalParameters  NCopyVariant=Disabled  FilterICVariant=InternalICsFilter  IntegratorICVariant=InternalICs  ExternalResetVariant=Disabled  TRSumVariant=Passthrough  SumFdbkVariant=Disabled  SumVariant=Sum_PID  TsampFilterVariant=InternalTs  TsampNgainVariant=Passthrough  TsampIntegralVariant=Disabled_SignalSpec  ExternalSaturationOutDataTypeStr=Inherit: Same as second input
  PID Controller3 : slpidlib/PID Controller  Controller=PID  Form=Parallel  TimeDomain=Continuous-time  UseExternalTs=off  SampleTime=-1  IntegratorMethod=Forward Euler  FilterMethod=Forward Euler  ControllerParametersSource=internal  P=4500  I=800  UseKiTs=off  D=8000  N=100  UseFilter=on  TunerSelectOption=Transfer Function Based (PID Tuner App)  InitialConditionSource=internal  InitialConditionForIntegrator=0  InitialConditionForFilter=0  DifferentiatorICPrevScaledInput=0  ExternalReset=none  TrackingMode=off  Kt=1  LimitOutput=off  SatLimitsSource=internal  UpperSaturationLimit=1  LowerSaturationLimit=-1  LinearizeAsGain=on  AntiWindupMode=none  Kb=1  LimitIntegrator=off  UpperIntegratorSaturationLimit=inf  LowerIntegratorSaturationLimit=-inf  POutMin=[]  POutMax=[]  IOutMin=[]  IOutMax=[]  DOutMin=[]  DOutMax=[]  NOutMin=[]  NOutMax=[]  SumOutMin=[]  SumOutMax=[]  SaturationOutMin=[]  SaturationOutMax=[]  PParamMin=[]  PParamMax=[]  IParamMin=[]  IParamMax=[]  DParamMin=[]  DParamMax=[]  NParamMin=[]  NParamMax=[]  KbParamMin=[]  KbParamMax=[]  KtParamMin=[]  KtParamMax=[]  KbOutMin=[]  KbOutMax=[]  KtOutMin=[]  KtOutMax=[]  IntegratorOutMin=[]  IntegratorOutMax=[]  FilterOutMin=[]  FilterOutMax=[]  SumI1OutMin=[]  SumI1OutMax=[]  SumI2OutMin=[]  SumI2OutMax=[]  SumI3OutMin=[]  SumI3OutMax=[]  SumI4OutMin=[]  SumI4OutMax=[]  SumDOutMin=[]  SumDOutMax=[]  DifferentiatorOutMin=[]  DifferentiatorOutMax=[]  FilterDiffOutCoefMin=[]  FilterDiffOutCoefMax=[]  ReciprocalOutMin=[]  ReciprocalOutMax=[]  SumDenOutMin=[]  SumDenOutMax=[]  SumNumOutMin=[]  SumNumOutMax=[]  DivideOutMin=[]  DivideOutMax=[]  UdiffTsProdOutMin=[]  UdiffTsProdOutMax=[]  NTsProdOutMin=[]  NTsProdOutMax=[]  UintegralTsProdOutMin=[]  UintegralTsProdOutMax=[]  UngainTsProdOutMin=[]  UngainTsProdOutMax=[]  ClampingZeroOutDataTypeStr=Inherit: Inherit via back propagation  ClampingZeroOutMin=[]  ClampingZeroOutMax=[]  FilterDenConstantOutDataTypeStr=Inherit: Inherit via back propagation  FilterDenConstantOutMin=[]  FilterDenConstantOutMax=[]  PCopyOutDataTypeStr=Inherit: Inherit via back propagation  PCopyOutMin=[]  PCopyOutMax=[]  NCopyOutDataTypeStr=Inherit: Inherit via back propagation  NCopyOutMin=[]  NCopyOutMax=[]  IntegratorContinuousStateAttributes=''  IntegratorStateMustResolveToSignalObject=off  IntegratorRTWStateStorageClass=Auto  FilterContinuousStateAttributes=''  FilterStateMustResolveToSignalObject=off  FilterRTWStateStorageClass=Auto  ParallelPVariant=InternalParameters  IdealPVariant=Disabled  IVariant=InternalParameters  DVariant=InternalParameters  IntegratorVariant=Continuous  SatVariant=Disabled  AWVariant=Passthrough  PCopyVariant=Disabled  TRVariant=Disabled  FdbkBlocksVariant=Forward  IdealPFdbkVariant=Disabled  SatFdbkVariant=Disabled  DerivativeFilterVariant=ContFilter  NVariant=InternalParameters  NCopyVariant=Disabled  FilterICVariant=InternalICsFilter  IntegratorICVariant=InternalICs  ExternalResetVariant=Disabled  TRSumVariant=Passthrough  SumFdbkVariant=Disabled  SumVariant=Sum_PID  TsampFilterVariant=InternalTs  TsampNgainVariant=Passthrough  TsampIntegralVariant=Disabled_SignalSpec  ExternalSaturationOutDataTypeStr=Inherit: Same as second input
  Product : Product
  Saturation 6V1 : Saturate  UpperLimit=5  LowerLimit=-5
  Saturation 6V2 : Saturate  UpperLimit=5  LowerLimit=-5
  Saturation 6V3 : Saturate  UpperLimit=5  LowerLimit=-5
  Scope : Scope
  Scope1 : Scope
  Scope2 : Scope
  Step : Step  Time=0  SampleTime=0
  magTorqueMatrix : Outport
  momentoDipolar : Outport  Port=2
  wires:
  Demux/3 -> PID Controller3/1, PID Controller20/1, PID Controller2/1
  Step/1 -> Product/2
  Campo Geomagnético1/1 -> Product/1
  Cross Product2/1 -> Add/3  "MgtZ"
  Mgt_ejeZ/1 -> Cross Product2/1
  Momento Dipolar Z/1 -> Mgt_ejeZ/1
  Saturation 6V3/1 -> Momento Dipolar Z/1  "PWR_mgt Y"
  PID Controller2/1 -> Manual Switch2/1
  Manual Switch2/1 -> Saturation 6V3/1
  MATLAB Function/2(momentoDipolar) -> Contribucion de cada Mgt2/2
  Add1/1 -> momentoDipolar/1, Contribucion de cada Mgt2/1
  MATLAB Function/1(magTorqueMatrix) -> Contribucion de cada Mgt1/2
  Add/1 -> magTorqueMatrix/1, Scope/1, Contribucion de cada Mgt1/1
  Cross Product1/1 -> Add/2, Contribucion de cada Mgt/2  "MgtY"
  Mgt_ejeY/1 -> Cross Product1/1, Add1/2
  Momento Dipolar Y/1 -> Mgt_ejeY/1
  Saturation 6V2/1 -> Momento Dipolar Y/1, MATLAB Function/3(voltageY), Scope2/1  "PWR_mgt Y"
  Cross Product/1 -> Contribucion de cada Mgt/1, Add/1  "MgtX"
  Mgt_ejeX/1 -> Cross Product/1, Add1/1
  Momento Dipolar X/1 -> Mgt_ejeX/1
  Manual Switch1/1 -> Saturation 6V1/1
  Constant1/1 -> Manual Switch1/1
  Constant/1 -> Manual Switch/2, MATLAB Function/4(voltageZ), Manual Switch2/2
  PID Controller20/1 -> Manual Switch/1
  Manual Switch/1 -> Saturation 6V2/1
  Product/1 -> Cross Product/2, Cross Product1/2, Cross Product2/2, MATLAB Function/1(B)
  Hz_error/1 -> Demux/1
  Saturation 6V1/1 -> Momento Dipolar X/1, MATLAB Function/2(voltageX), Scope1/1  "PWR_mgt X"
  PID Controller3/1 -> Manual Switch1/2

== matlab function LinearModelClosedLoopTest_RW_and_Mgt_models/Non Linear SC Dynamics/MATLAB Function ==
  data: Td input; Mgt output; Mgt input
function Mgt = fcn(Td,Mgt)

    if (Td(3)<0)
        Mgt = abs(Mgt);
    else
        Mgt = -Mgt;
    end

end

== matlab function LinearModelClosedLoopTest_RW_and_Mgt_models/MATLAB Function ==
  data: H_error input; B input; H_error output
function H_error = fcn(H_error,B)

if (B(1)> 0)
    HGain =-1;
else
    HGain = 1;

end
H_error = H_error*HGain; 
end

== matlab function LinearModelClosedLoopTest_RW_and_Mgt_models/Subsystem1/MATLAB Function ==
  data: B input; magTorqueMatrix output; voltageX input; voltageY input; voltageZ input; momentoDipolar output
function [magTorqueMatrix,momentoDipolar] = magTorqueFunction(B,voltageX,voltageY,voltageZ)

%d = 1.45e-2; % Diametro mgt [m]
d = 1.45e-2; % Diametro mgt [m]
A =d^2*pi/4;

%n=sqrt(L*l/(mu_0*mu_r*A)); % # Vueltas 
n = 5412;

%R = 50.7 ;% Resistencia mgt [Ohm];
R = 30 ;% Resistencia mgt [Ohm];
ix = voltageX/R;
iy = voltageY/R;
iz = voltageZ/R;

% M = [n*ix*A n*iy*A n*iz*A]';
% 
% magTorqueMatrix = -skew(B)*M;

magTorqueMatrix_X = cross(n*ix*A*[1 0 0],B);
magTorqueMatrix_Y = cross(n*iy*A*[0 1 0],B);
magTorqueMatrix_Z = cross(n*iz*A*[0 0 1],B);
 momentoDipolar = [n*ix*A n*iy*A n*iz*A];

magTorqueMatrix = magTorqueMatrix_X+magTorqueMatrix_Y+magTorqueMatrix_Z;

== matlab function LinearModelClosedLoopTest_RW_and_Mgt_models/Non Linear SC Dynamics/MATLAB Function1 ==
  data: cubeSatOmega input; q_dot output; q input
function q_dot = omega2qdot(cubeSatOmega,q)

wx = cubeSatOmega(1);
wy = cubeSatOmega(2);
wz = cubeSatOmega(3);

OmegaMatrix = [0 wz -wy wx ;
               -wz 0 wx wy; 
               wy -wx 0 wz;
               -wx -wy -wz 0];
            
q_dot=0.5*OmegaMatrix*q;

end

== matlab function LinearModelClosedLoopTest_RW_and_Mgt_models/MATLAB Function1 ==
  data: signal input; B input; signal output
function signal = fcn(signal,B)

if (B(2)> 0)
    HGain =1;
else
    HGain = -1;

end
signal = signal*HGain; 
end
